simulink model "cruise_control_dut"  (R2014b)
settings: Solver=FixedStepDiscrete  StartTime=0  StopTime=0.069999999999999993  FixedStep=0.01  RelTol=1e-3
settings Model: SldvGeneratedHarnessModel=TestUnitModel=cosim_cruise_control|  CovMetricSettings=dcmoe  CovHTMLOptions=-sRT=1 -aTS=1 -bRG=1 -bTC=0 -hTR=0 -nFC=0 -scm=1 -bcm=1 -xEv=0  covSaveCumulativeToWorkspaceVar=off  CovSaveSingleToWorkspaceVar=off  CovReportOnPause=off  CovModelRefEnable=off  Creator=The MathWorks Inc.  LastModifiedBy=kotsuka
settings DataIOCC: SaveFormat=StructureWithTime  SignalLoggingSaveFormat=ModelDataLogs
settings OptimizationCC: BlockReduction=off  ConditionallyExecuteInputs=off  InlineParams=on  InlineInvariantSignals=on  ExpressionFolding=off  ExpressionDepthLimit=2147483647  InitFltsAndDblsToZero=on  EfficientMapNaN2IntZero=off
settings DebuggingCC: SaveWithParameterizedLinksMsg=none  UnderspecifiedInitializationDetection=Classic  MergeDetectMultiDrivingBlocksExec=none  SignalResolutionControl=TryResolveAllWithWarning  InheritedTsInSrcMsg=none  FcnCallInpInsideContextMsg=UseLocalSettings  StateNameClashWarn=warning  StrictBusMsg=Warning
settings GRTTargetCC: TargetFcnLib=ansi_tfl_tmw.mat  CombineOutputUpdateFcns=off  GRTInterface=on
settings ConfigComp: Description=Design Verifier Custom Configuration Component  DVMaxProcessTime=60  DVMakeOutputFilesUnique=off  DVParameters=on  DVModelCoverageObjectives=MCDC  DVMaxTestCaseSteps=500  DVTestSuiteOptimization=CombinedObjectives  DVAssertions=EnableAll  DVProofAssumptions=EnableAll  DVCovFilter=on  DVDetectActiveLogic=on  DVProvingStrategy=FindViolation

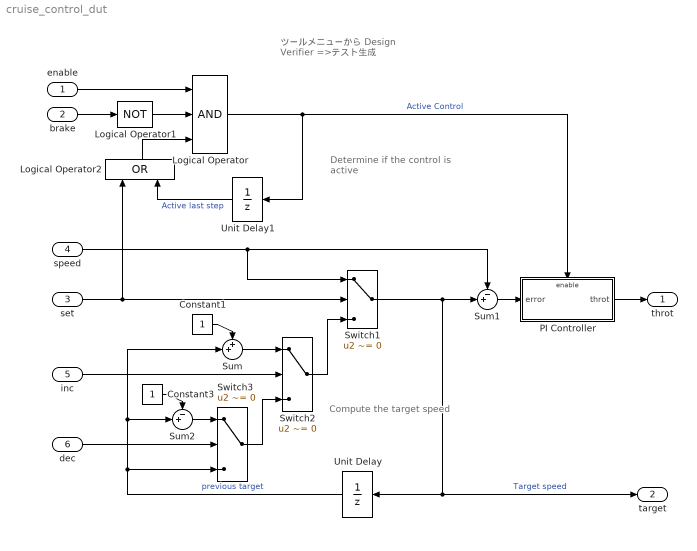
== system cruise_control_dut ==
  note: Compute the
      | target speed
  note: Determine if the
      | control is active
  note: ツールメニューから
      | Design Verifier
      | =>テスト生成
  enable : Inport  OutDataTypeStr=boolean
  brake : Inport  Port=2  OutDataTypeStr=boolean
  set : Inport  Port=3  OutDataTypeStr=boolean
  speed : Inport  Port=4  OutDataTypeStr=double
  inc : Inport  Port=5  OutDataTypeStr=boolean
  dec : Inport  Port=6  OutDataTypeStr=boolean
  Constant1 : Constant
  Constant3 : Constant
  Logical Operator : Logic  Inputs=3  AllPortsSameDT=off  OutDataTypeStr=boolean
  Logical Operator1 : Logic  Operator=NOT  AllPortsSameDT=off  OutDataTypeStr=boolean
  Logical Operator2 : Logic  Operator=OR  AllPortsSameDT=off  OutDataTypeStr=boolean
  PI Controller : Subsystem
  Sum : Sum  Inputs=++|
  Sum1 : Sum  Inputs=-+|
  Sum2 : Sum  Inputs=-+|
  Switch1 : Switch  Criteria=u2 ~= 0
  Switch2 : Switch  Criteria=u2 ~= 0
  Switch3 : Switch  Criteria=u2 ~= 0
  Unit Delay : UnitDelay  SampleTime=0.01
  Unit Delay1 : UnitDelay  SampleTime=0.01
  throt : Outport
  target : Outport  Port=2
  wires:
  PI Controller/1(throt) -> throt/1
  Sum1/1 -> PI Controller/1(error)
  Logical Operator/1 -> PI Controller/Enable, Unit Delay1/1  "Active Control"
  Unit Delay1/1 -> Logical Operator2/2  "Active last step"
  Logical Operator2/1 -> Logical Operator/3
  Switch1/1 -> Sum1/2, target/1, Unit Delay/1  "Target speed"
  Unit Delay/1 -> Switch3/3, Sum2/2, Sum/2  "previous target"
  Switch3/1 -> Switch2/3
  Switch2/1 -> Switch1/3
  Sum2/1 -> Switch3/1
  Constant3/1 -> Sum2/1
  dec/1 -> Switch3/2
  Sum/1 -> Switch2/1
  Constant1/1 -> Sum/1
  inc/1 -> Switch2/2
  speed/1 -> Switch1/1, Sum1/1
  set/1 -> Logical Operator2/1, Switch1/2
  Logical Operator1/1 -> Logical Operator/2
  enable/1 -> Logical Operator/1
  brake/1 -> Logical Operator1/1

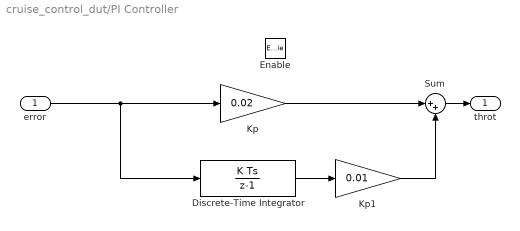
== system cruise_control_dut/PI Controller ==
  error : Inport
  Enable : EnablePort
  Discrete-Time Integrator : DiscreteIntegrator  SampleTime=0.01  LimitOutput=on  UpperSaturationLimit=5  LowerSaturationLimit=-5
  Kp : Gain  Gain=0.02
  Kp1 : Gain  Gain=0.01
  Sum : Sum  Inputs=|++
  throt : Outport  InitialOutput=0
  wires:
  Sum/1 -> throt/1
  error/1 -> Discrete-Time Integrator/1, Kp/1
  Discrete-Time Integrator/1 -> Kp1/1
  Kp1/1 -> Sum/2
  Kp/1 -> Sum/1
